simulink model "PARALELO"  (R2023a)
settings: Solver=VariableStepAuto  StartTime=0.0  StopTime=2/Frequency  RelTol=1e-3
undefined symbols (not defined in the file): C, Frequency, L, R, V
libraries: spsSeriesRLCBranchLib x4, spsFourierLib x4, spsCurrentMeasurementLib x1, spsMultimeterLib x1, spsACVoltageSourceLib x1, sps_lib x1
settings Model: Creator=XIOMARA  LastModifiedBy=XIOMARA

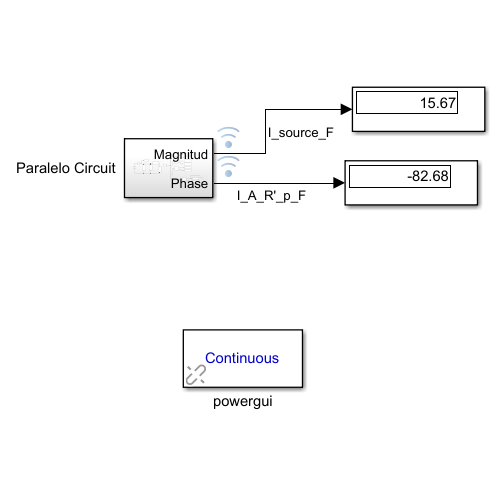
[thumbnail: Simulink's stored preview of the top-level diagram]
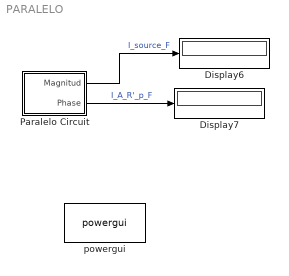
== system PARALELO ==
  Display6 : Display
  Display7 : Display
  Paralelo Circuit : Subsystem
  powergui : sps_lib/powergui  Priority=1  SimulationMode=Continuous  SampleTime=50e-6  frequency=60  Iterations=50  frequencyindice=10000  Pbase=100e6  ErrMax=1e-4  UnitsV=kV  UnitsW=MW  buscounter=0  FunctionMessages=off  echomessages=off  EnableUseOfTLC=off  CurrentSourceSwitches=off  DisableSnubberDevices=off  DisableRonSwitches=off  DisableVfSwitches=off  DisplayEquations=off  AutomaticDiscreteSolvers=off  SolverType=Tustin/Backward Euler (TBE)  Interpol=off  ExternalGateDelay=off  methode=off  Ts=100  x0status=blocks  SPID=on  SwTol=0  HookPort=off  NonlinearTolerance=1e-4  nMaxIteration=100  ContinueOnMaxIteration=off  RestoreLinks=warning  ResistiveCurrentMeasurement=off  Frange=[0:2:500]  Ylog=off  Xlog=on  ShowGrid=off  save=off  variable=ZData  structure=0  ZoomFFT=off  StartTime=0.0  cycles=1  DisplayStyle=1  fundamental=60  FreqAxis=off  MaxFrequency=1000  frequencyindicesteady=1  RmsSteady=1  display=off
  wires:
  Paralelo Circuit/1(Magnitud) -> Display6/1  "I_source_F"
  Paralelo Circuit/2(Phase) -> Display7/1  "I_A_R'_p_F"

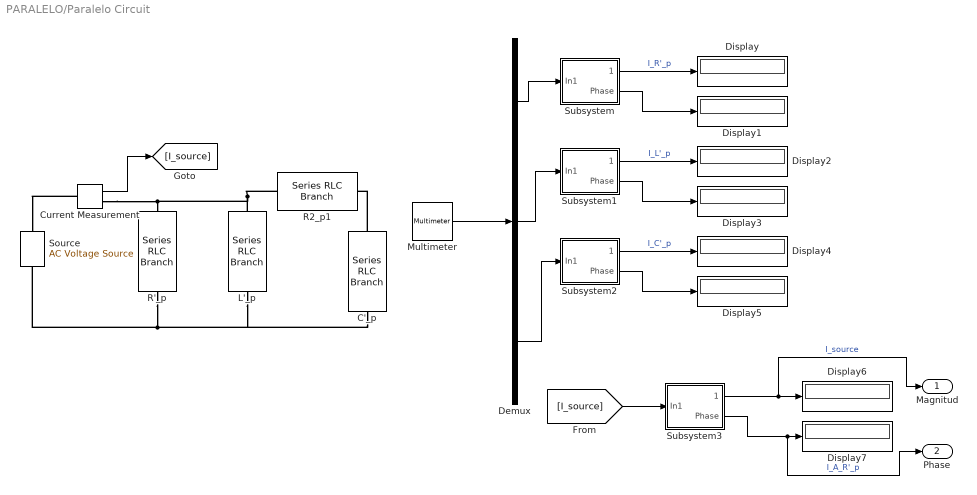
== system PARALELO/Paralelo Circuit ==
  "C'_p " : spsSeriesRLCBranchLib/Series RLC Branch  LConnTagsString=__new0  RConnTagsString=__new0  BranchType=C  Resistance=1  Inductance=C  SetiL0=off  InitialCurrent=0  Capacitance=C  Setx0=off  InitialVoltage=0  Measurements=Branch current
  Current Measurement : spsCurrentMeasurementLib/Current Measurement  PhasorSimulation=off  OutputType=Complex  PSBequivalent=0
  Demux : Demux  Outputs=3
  Display{,1..7} (8 alike) : Display
  L'_p : spsSeriesRLCBranchLib/Series RLC Branch  LConnTagsString=__new0  RConnTagsString=__new0  BranchType=L  Resistance=1  Inductance=L  SetiL0=off  InitialCurrent=0  Capacitance=1e-6  Setx0=off  InitialVoltage=0  Measurements=Branch current
  Multimeter : spsMultimeterLib/Multimeter  L=3  sel=[3 2 1]  yselected={}  Gain=[1 1 1]  OutputType=Complex  PlotAtSimulationStop=off  PhasorSimulation=off
  R'_p : spsSeriesRLCBranchLib/Series RLC Branch  LConnTagsString=__new0  RConnTagsString=__new0  BranchType=R  Resistance=R  Inductance=L  SetiL0=off  InitialCurrent=0  Capacitance=1e-6  Setx0=off  InitialVoltage=0  Measurements=Branch current
  R2_p1 : spsSeriesRLCBranchLib/Series RLC Branch  LConnTagsString=__new0  RConnTagsString=__new0  BranchType=R  Resistance=1e-6  Inductance=1e-3  SetiL0=off  InitialCurrent=0  Capacitance=1e-6  Setx0=off  InitialVoltage=0  Measurements=None
  Source : spsACVoltageSourceLib/AC Voltage Source  Amplitude=V*sqrt(2)  Phase=0  Frequency=Frequency  SampleTime=0  Measurements=None  BusType=swing  Pref=10e3  Qref=0  Qmin=-inf  Qmax=+inf
  Subsystem : Subsystem
  Subsystem1 : Subsystem
  Subsystem2 : Subsystem
  Subsystem3 : Subsystem
  Magnitud : Outport
  Phase : Outport  Port=2
  wires:
  Multimeter/1 -> Demux/1
  Demux/1 -> Subsystem/1(In1)
  Subsystem/1(Magnitud) -> Display/1  "I_R'_p"
  Subsystem/2(Phase) -> Display1/1
  Demux/2 -> Subsystem1/1(In1)
  Subsystem1/1(Magnitud) -> Display2/1  "I_L'_p"
  Subsystem1/2(Phase) -> Display3/1
  Demux/3 -> Subsystem2/1(In1)
  Subsystem2/1(Magnitud) -> Display4/1  "I_C'_p"
  Subsystem2/2(Phase) -> Display5/1
  Current Measurement/1 -> [I_source]
  Subsystem3/2(Phase) -> Phase/1, Display7/1  "I_A_R'_p"
  Subsystem3/1(Magnitud) -> Magnitud/1, Display6/1  "I_source"
  [I_source] -> Subsystem3/1(In1)
  connections:
  R'_p/RConn1 -- "C'_p "/RConn1 -- L'_p/RConn1 -- Source/LConn1
  L'_p/LConn1 -- Current Measurement/RConn1 -- R'_p/LConn1 -- R2_p1/LConn1
  "C'_p "/LConn1 -- R2_p1/RConn1
  Current Measurement/LConn1 -- Source/RConn1

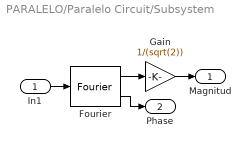
== system PARALELO/Paralelo Circuit/Subsystem ==
  In1 : Inport
  Fourier : spsFourierLib/Fourier  Freq=Frequency  n=1  InInit=[0, 0]  Ts=0
  Gain : Gain  Gain=1/(sqrt(2))
  Magnitud : Outport
  Phase : Outport  Port=2
  wires:
  Fourier/1 -> Gain/1
  Fourier/2 -> Phase/1
  Gain/1 -> Magnitud/1
  In1/1 -> Fourier/1

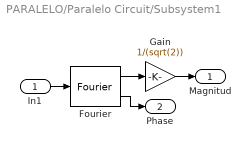
== system PARALELO/Paralelo Circuit/Subsystem1 ==
  In1 : Inport
  Fourier : spsFourierLib/Fourier  Freq=Frequency  n=1  InInit=[0, 0]  Ts=0
  Gain : Gain  Gain=1/(sqrt(2))
  Magnitud : Outport
  Phase : Outport  Port=2
  wires:
  Fourier/1 -> Gain/1
  Fourier/2 -> Phase/1
  Gain/1 -> Magnitud/1
  In1/1 -> Fourier/1

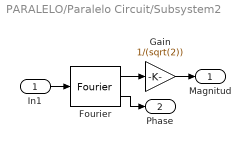
== system PARALELO/Paralelo Circuit/Subsystem2 ==
  In1 : Inport
  Fourier : spsFourierLib/Fourier  Freq=Frequency  n=1  InInit=[0, 0]  Ts=0
  Gain : Gain  Gain=1/(sqrt(2))
  Magnitud : Outport
  Phase : Outport  Port=2
  wires:
  Fourier/1 -> Gain/1
  Fourier/2 -> Phase/1
  Gain/1 -> Magnitud/1
  In1/1 -> Fourier/1

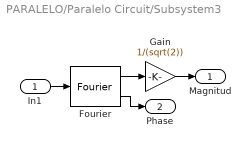
== system PARALELO/Paralelo Circuit/Subsystem3 ==
  In1 : Inport
  Fourier : spsFourierLib/Fourier  Freq=Frequency  n=1  InInit=[0, 0]  Ts=0
  Gain : Gain  Gain=1/(sqrt(2))
  Magnitud : Outport
  Phase : Outport  Port=2
  wires:
  Fourier/1 -> Gain/1
  Fourier/2 -> Phase/1
  Gain/1 -> Magnitud/1
  In1/1 -> Fourier/1
